simulink model "LaneFollowingTestBenchExample"  (R2023a)
settings: Solver=VariableStepAuto  StartTime=0.0  StopTime=simStopTime  RelTol=1e-3
PostLoadFcn:
  | if exist('scenarioName','var')
  |   helperLFSetUp(scenarioName)
  | else
  |   helperLFSetUp()
  | end
values from neighbouring files (symbols this model uses):
  Ts = 0.01    [Working.m]    (also in Working_flipped.m)
  v_set = 15    [helperLFSetUp.m]
undefined symbols (not defined in the file or in its folder): driving, egoCarID, lr, m, matlabshared, tau
libraries: drivingscenarioandsensors x6, trackingutilitieslib x1, autolibshared x1
CloseFcn:
  | helperLFCleanUp
settings Model: Creator=The MathWorks, Inc.  LastModifiedBy=Administrator
settings SolverCC: AlgebraicLoopSolver=TrustRegion
settings DataIOCC: ReturnWorkspaceOutputs=off
settings DebuggingCC: ParameterPrecisionLossMsg=none  UnconnectedInputMsg=warning  UnconnectedOutputMsg=warning  UnconnectedLineMsg=warning  PregeneratedLibrarySubsystemCodeDiagnostic=none  ArithmeticOperatorsInVariantConditions=warning
settings HardwareCC: ProdLongLongMode=on
settings ModelReferenceCC: EnableRefExpFcnMdlSchedulingChecks=on
settings SFSimCC: SimUseLocalCustomCode=off
settings RTWCC: GenerateReport=on  RTWUseLocalCustomCode=off  LaunchReport=on  DLArmComputeVersion=19.05
settings ConfigComp: CovScope=ReferencedModels  CovIncludeTopModel=off

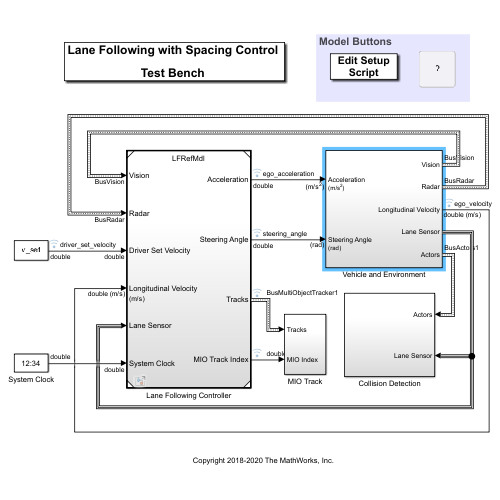
[thumbnail: Simulink's stored preview of the top-level diagram]
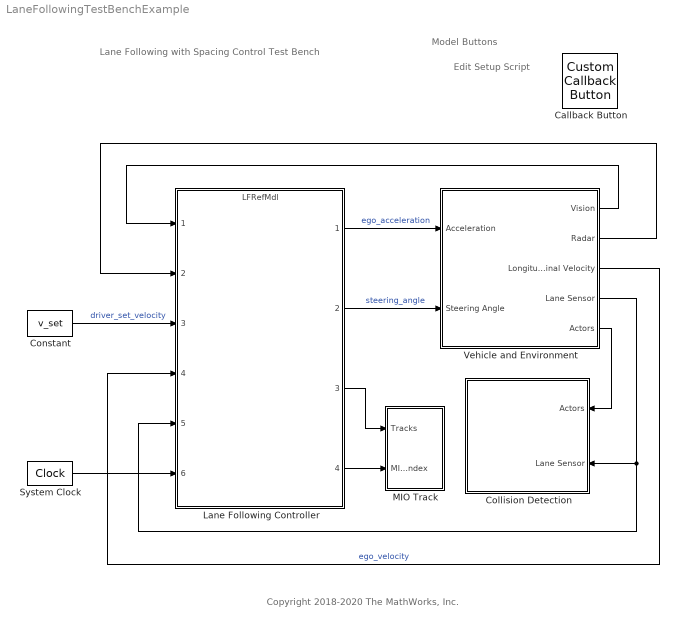
== system LaneFollowingTestBenchExample ==
  note: Copyright 2018-2020 The MathWorks, Inc.
  note: Edit Setup Script
  note: Lane Following with Spacing Control
      | Test Bench
  note: Model Buttons
  Callback Button : CustomCallbackButton  Configuration="{\"components\":[{\"name\":\"BackgroundImageComponent\",\"settings\":{\"image\":{\"size\":[0,0],\"src\":\"default\",\"srcOrientation\":\"Right\"},\"position\":[0,0,1,1]}},{\"name\":\"ButtonStateComponent\",\"settings\":{\"buttonType\":\"momentary\",\"clickFcn\":\"exampleName = 'lane-following-control-with-sensor-fusion-and-lane-detection.html';\\nif license('test','automated_driving_toolbox') && ~isempty(ver('driving'))\\n   web(fullfile(docroot,'driving','ug', exampleName));\\nelseif license('test','MPC_Toolbox') && ~isempty(ver('mpc'))\\n    web(fullfile(docroot,'mpc','ug', exampleName));\\nelse\\n    web(fullfile('https:\\/\\/www.mathworks.com\\/help','driving','ug',exampleName));\\nend\",\"onValue\":1,\"position\":[0,0,1,1],\"pressDelay\":\"500\",\"pressFcn\":\"\",\"repeatInterval\":\"0\",\"states\":[{\"horizontalAlignment\":\"center\",\"image\":{\"position\":[0,0,1,1],\"src\":\"default\",\"srcOrientation\":\"Right\"},\"label\":{\"color\":[0.01176470588,0.01176470588,0.01176470588,1],\"icon\":{\"size\":[0,0],\"src\":\"default\",\"srcOrientation\":\"Right\"},\"iconPlacement\":\"left\",\"text\":{\"content\":\"?\"}},\"labelOffset\":[0,0],\"verticalAlignment\":\"middle\"},{\"horizontalAlignment\":\"center\",\"image\":{\"position\":[0,0,1,1],\"src\":\"default\",\"srcOrientation\":\"Right\"},\"label\":{\"color\":[0.01176470588,0.01176470588,0.01176470588,1],\"icon\":{\"size\":[0,0],\"src\":\"default\",\"srcOrientation\":\"Right\"},\"iconPlacement\":\"left\",\"text\":{\"content\":\"?\"}},\"labelOffset\":[0,0],\"verticalAlignment\":\"middle\"},{\"horizontalAlignment\":\"center\",\"image\":{\"position\":[0,0,1,1],\"src\":\"default\",\"srcOrientation\":\"Right\"},\"label\":{\"color\":[0.01176470588,0.01176470588,0.01176470588,1],\"icon\":{\"size\":[0,0],\"src\":\"default\",\"srcOrientation\":\"Right\"},\"iconPlacement\":\"left\",\"text\":{\"content\":\"?\"}},\"labelOffset\":[0,0],\"verticalAlignment\":\"middle\"},{\"horizontalAlignment\":\"center\",\"image\":{\"position\":[0,0,1,1],\"src\":\"default\",\"srcOrientation\":\"Right\"},\"label\":{\"color\":[0.01176470588,0.01176470588,0.01176470588,1],\"icon\":{\"size\":[0,0],\"src\":\"default\",\"srcOrientation\":\"Right\"},\"iconPlacement\":\"left\",\"text\":{\"content\":\"?\"}},\"labelOffset\":[0,0],\"verticalAlignment\":\"middle\"}]}},{\"name\":\"ForegroundImageComponent\",\"settings\":{\"image\":{\"size\":[0,0],\"src\":\"default\",\"srcOrientation\":\"Right\"},\"isForeground\":1,\"position\":[0,0,1,1]}}],\"settings\":{\"BindingType\":\"standalone\",\"backgroundColor\":[244,244,244,1],\"backgroundOffset\":0.2,\"backgroundOpacity\":1,\"fixedAspectRatio\":\"off\",\"foregroundColor\":[0.01176470588,0.01176470588,0.01176470588,1],\"migratedFromLegacy\":true,\"useBackgroundColor\":true,\"variant\":\"callback\",\"version\":\"R2023a\"},\"type\":\"Button\"}"  CustomBackgroundColor="{\"color\":[0.9568627451,0.9568627451,0.9568627451],\"show\":true}"
  Collision Detection : Subsystem
  Constant : Constant  Value=v_set  SampleTime=Ts
  Lane Following Controller : ModelReference  ModelNameDialog=LFRefMdl  SimulationMode=Normal  CodeInterface=Top model  ModelReferenceVersion=6.1
  MIO Track : Subsystem
  System Clock : DigitalClock  SampleTime=Ts
  Vehicle and Environment : Subsystem
  wires:
  Lane Following Controller/1 -> Vehicle and Environment/1(Acceleration)  "ego_acceleration"
  Lane Following Controller/2 -> Vehicle and Environment/2(Steering Angle)  "steering_angle"
  Constant/1 -> Lane Following Controller/3  "driver_set_velocity"
  Vehicle and Environment/3(Longitudinal Velocity) -> Lane Following Controller/4  "ego_velocity"
  Vehicle and Environment/4(Lane Sensor) -> Lane Following Controller/5, Collision Detection/2(Lane Sensor)
  Vehicle and Environment/2(Radar) -> Lane Following Controller/2
  Vehicle and Environment/1(Vision) -> Lane Following Controller/1
  Lane Following Controller/3 -> MIO Track/1(Tracks)
  Lane Following Controller/4 -> MIO Track/2(MIO Index)
  Vehicle and Environment/5(Actors) -> Collision Detection/1(Actors)
  System Clock/1 -> Lane Following Controller/6

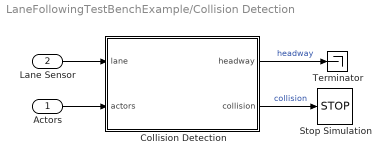
== system LaneFollowingTestBenchExample/Collision Detection ==
  Actors : Inport
  Lane Sensor : Inport  Port=2
  Collision Detection : MATLAB Function  TreatAsAtomicUnit=on
  Stop Simulation : Stop
  Terminator : Terminator
  wires:
  Collision Detection/2(collision) -> Stop Simulation/1  "collision"
  Actors/1 -> Collision Detection/2(actors)
  Lane Sensor/1 -> Collision Detection/1(lane)
  Collision Detection/1(headway) -> Terminator/1  "headway"

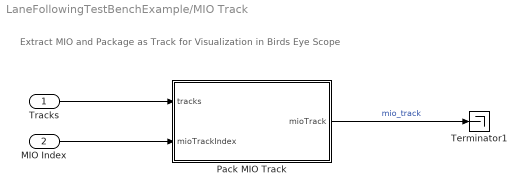
== system LaneFollowingTestBenchExample/MIO Track ==
  note: Extract MIO and Package as Track for Visualization in Birds Eye Scope
  Tracks : Inport
  MIO Index : Inport  Port=2
  Pack MIO Track : MATLAB Function  TreatAsAtomicUnit=on
  Terminator1 : Terminator
  wires:
  Tracks/1 -> Pack MIO Track/1(tracks)
  Pack MIO Track/1(mioTrack) -> Terminator1/1  "mio_track"
  MIO Index/1 -> Pack MIO Track/2(mioTrackIndex)

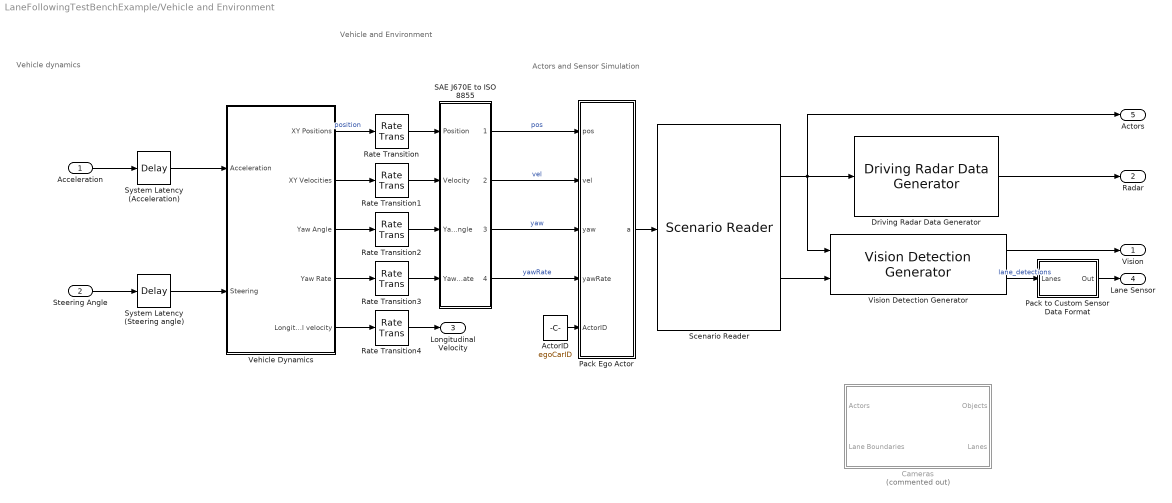
== system LaneFollowingTestBenchExample/Vehicle and Environment ==
  note: Vehicle dynamics
  note: Actors and Sensor Simulation
  note: Vehicle and Environment
  Acceleration : Inport  Unit=m/s^2
  Steering Angle : Inport  Port=2  Unit=rad
  ActorID : Constant  Value=egoCarID
  Cameras : Subsystem  Commented=on
  Driving Radar Data Generator : drivingscenarioandsensors/Driving Radar Data Generator  SensorIndex=2  UpdateRate=10  MountingLocation=[ 3.7, 0, 0.2 ]  MountingAngles=[0 0 0]  HasElevation=off  HasRangeRate=on  HasNoise=on  HasFalseAlarms=on  HasOcclusion=on  MaxNumReportsSource=Property  MaxNumReports=50  TargetReportFormat=Clustered detections  DetectionCoordinates=Body  TrackCoordinates=Body  BusNameSource=Property  BusName=BusRadar  AzimuthResolution=4  ElevationResolution=5  RangeResolution=2.5  RangeRateResolution=0.5  AzimuthBiasFraction=0.1  ElevationBiasFraction=0.1  RangeBiasFraction=0.05  RangeRateBiasFraction=0.05  FieldOfView=[ 20, 5 ]  RangeLimits=[ 0, 174 ]  RangeRateLimits=[ -100, 100 ]  DetectionProbability=0.9  FalseAlarmRate=1e-06  ReferenceRange=100  ReferenceRCS=0  CenterFrequency=77e9  FilterInitializationFcn=initcvekf  ConfirmationThreshold=[2 3]  DeletionThreshold=[5 5]  InitialSeedSource=Repeatable  InitialSeed=0  UsedSeed=matlabshared.tracking.internal.SimulinkUtilities.seedManager(gcb)  ProfilesSource=From Scenario Reader block  ProfilesParameters=driving.internal.ActorProfilesRadarParameters  ProfilesExpression=struct('ClassID',0,'Length',4.7,'Width',1.8,'Height',1.4,'OriginOffset',[-1.35 0 0],'RCSPattern',[10 10;10 10],'RCSAzimuthAngles',[-180 180],'RCSElevationAngles',[-90 90])
  Pack Ego Actor : MATLAB Function  TreatAsAtomicUnit=on
  Pack to Custom Sensor Data Format : Subsystem
  Rate Transition{,1..4} (5 alike) : RateTransition  OutPortSampleTime=Ts
  SAE J670E to ISO 8855 : Subsystem
  Scenario Reader : drivingscenarioandsensors/Scenario Reader  ScenarioSource=From workspace  ScenarioFileName=LFACC_04_Curve_CutInOut.mat  ScenarioVariableName=scenario  OutputCoordinateSystem=Vehicle coordinates  EgoVehicleSource=Input port  EgoVehicleActorID=egoCarID  OrientVehiclesOnRoad=off  OutputEgoVehiclePose=off  OutputEgoVehicleState=off  SampleTime=0.1  LaneBoundaryOutput=Ego vehicle lane boundaries  LaneBoundaryDistance=0:0.5:60  LaneBoundaryLocation=Inner edge of lane markings  BusNameSource=Auto  BusName=BusActors  BusNumActorsSource=Scenario  BusNumActors=100  BusName2Source=Auto  BusName2=BusLaneBoundaries  BusNumLaneBoundariesSource=Scenario  BusNumLaneBoundaries=10  BusName3Source=Auto  BusName3=BusEgoActor  BusName4Source=Auto  BusName4=BusEgoState  ShowCoordinateLabels=on  SimulateUsing=Interpreted execution
  System Latency (Acceleration) : TransportDelay  DelayTime=Ts
  System Latency (Steering angle) : TransportDelay  DelayTime=Ts
  Vehicle Dynamics : Subsystem  VariantControl=Variant2
  Vision Detection Generator : drivingscenarioandsensors/Vision Detection Generator  SensorIndex=1  DetectorOutput=Lanes and objects  UpdateInterval=0.1  LaneUpdateInterval=0.1  SensorLocation=[ 1.9, 0 ]  Height=1.1  Yaw=0  Pitch=1  Roll=0  BusNameSource=Property  BusName=BusVision  BusName2Source=Property  BusName2=BusLanes  MaxNumDetectionsSource=Property  MaxNumDetections=20  MaxNumLanesSource=Property  MaxNumLanes=2  DetectionCoordinates=Ego Cartesian  SimulateUsing=Interpreted execution  MaxRange=150  BoundingBoxAccuracy=5  ProcessNoiseIntensity=5  MaxSpeed=50  MaxAllowedOcclusion=0.5  MinObjectImageSize=[ 10, 10 ]  DetectionProbability=0.9  FalsePositivesPerImage=0.1  MinLaneImageSize=[ 20, 3 ]  LaneBoundaryAccuracy=3  HasNoise=on  InitialSeedSource=Repeatable  InitialSeed=0  UsedSeed=driving.internal.SimulinkUtilities.seedManager(gcb)  ActorProfilesSource=From Scenario Reader block  ActorProfilesParameters=driving.internal.ActorProfilesParameters  ActorProfilesExpression=struct( 'ClassID', 0, 'Length', 4.7, 'Width', 1.8, 'Height', 1.4, 'OriginOffset', [ -1.35, 0, 0 ] )  Intrinsics=driving.internal.cameraIntrinsics('FocalLength',[ 600,600 ])
  Vision : Outport  VectorParamsAs1DForOutWhenUnconnected=off
  Radar : Outport  Port=2  VectorParamsAs1DForOutWhenUnconnected=off
  Longitudinal Velocity : Outport  Port=3  VectorParamsAs1DForOutWhenUnconnected=off
  Lane Sensor : Outport  Port=4  VectorParamsAs1DForOutWhenUnconnected=off
  Actors : Outport  Port=5  VectorParamsAs1DForOutWhenUnconnected=off
  wires:
  Scenario Reader/1 -> Actors/1, Driving Radar Data Generator/1, Vision Detection Generator/1
  Vehicle Dynamics/2(XY Velocities) -> Rate Transition1/1
  Vehicle Dynamics/3(Yaw Angle) -> Rate Transition2/1
  Vehicle Dynamics/4(Yaw Rate) -> Rate Transition3/1
  Vehicle Dynamics/1(XY Positions) -> Rate Transition/1  "position"
  Pack to Custom Sensor Data Format/1(Out) -> Lane Sensor/1
  Rate Transition4/1 -> Longitudinal Velocity/1
  Vehicle Dynamics/5(Longitudinal velocity) -> Rate Transition4/1
  Scenario Reader/2 -> Vision Detection Generator/2
  Driving Radar Data Generator/1 -> Radar/1
  Pack Ego Actor/1(a) -> Scenario Reader/1
  Acceleration/1 -> System Latency (Acceleration)/1
  Steering Angle/1 -> System Latency (Steering angle)/1
  System Latency (Acceleration)/1 -> Vehicle Dynamics/1(Acceleration)
  System Latency (Steering angle)/1 -> Vehicle Dynamics/2(Steering)
  SAE J670E to ISO 8855/1(1) -> Pack Ego Actor/1(pos)  "pos"
  SAE J670E to ISO 8855/2(2) -> Pack Ego Actor/2(vel)  "vel"
  SAE J670E to ISO 8855/3(3) -> Pack Ego Actor/3(yaw)  "yaw"
  SAE J670E to ISO 8855/4(4) -> Pack Ego Actor/4(yawRate)  "yawRate"
  Rate Transition3/1 -> SAE J670E to ISO 8855/4(Yaw Rate)
  Rate Transition2/1 -> SAE J670E to ISO 8855/3(Yaw Angle)
  Rate Transition1/1 -> SAE J670E to ISO 8855/2(Velocity)
  Rate Transition/1 -> SAE J670E to ISO 8855/1(Position)
  ActorID/1 -> Pack Ego Actor/5(ActorID)
  Vision Detection Generator/2 -> Pack to Custom Sensor Data Format/1(Lanes)  "lane_detections"
  Vision Detection Generator/1 -> Vision/1

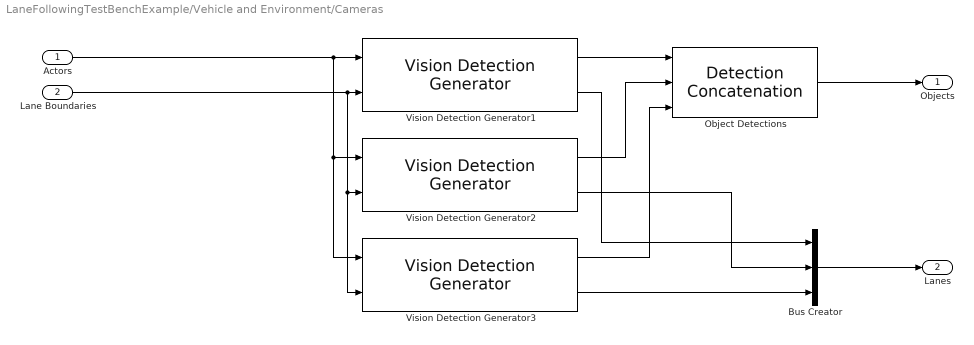
== system LaneFollowingTestBenchExample/Vehicle and Environment/Cameras ==
  Actors : Inport
  Lane Boundaries : Inport  Port=2
  Bus Creator : BusCreator  Inputs=3
  Object Detections : trackingutilitieslib/Detection Concatenation  NumInputs=3  BusNameSource=Auto  BusName=BusDetectionConcatenation  SimulateUsing=Interpreted execution
      settings: LibrarySourceBlock=drivinglib/Detection Concatenation
  Vision Detection Generator1 : drivingscenarioandsensors/Vision Detection Generator  SensorIndex=3  DetectorOutput=Lanes and objects  UpdateInterval=0.1  LaneUpdateInterval=0.1  SensorLocation=[ 1.835, 0 ]  Height=1.1  Yaw=0  Pitch=1  Roll=0  BusNameSource=Property  BusName=BusVision  BusName2Source=Property  BusName2=BusLanes  MaxNumDetectionsSource=Property  MaxNumDetections=20  MaxNumLanesSource=Property  MaxNumLanes=2  DetectionCoordinates=Ego Cartesian  SimulateUsing=Interpreted execution  MaxRange=150  BoundingBoxAccuracy=5  ProcessNoiseIntensity=5  MaxSpeed=50  MaxAllowedOcclusion=0.5  MinObjectImageSize=[ 10, 10 ]  DetectionProbability=0.9  FalsePositivesPerImage=0.1  MinLaneImageSize=[ 20, 3 ]  LaneBoundaryAccuracy=3  HasNoise=on  InitialSeedSource=Repeatable  InitialSeed=0  UsedSeed=driving.internal.SimulinkUtilities.seedManager(gcb)  ActorProfilesSource=From Scenario Reader block  ActorProfilesParameters=driving.internal.ActorProfilesParameters  ActorProfilesExpression=struct( 'ClassID', 0, 'Length', 4.7, 'Width', 1.8, 'Height', 1.4, 'OriginOffset', [ -1.35, 0, 0 ] )  Intrinsics=driving.internal.cameraIntrinsics('FocalLength',[ 800,800 ])
  Vision Detection Generator2 : drivingscenarioandsensors/Vision Detection Generator  SensorIndex=5  DetectorOutput=Lanes and objects  UpdateInterval=0.1  LaneUpdateInterval=0.1  SensorLocation=[2, 0.945]  Height=1.1  Yaw=90  Pitch=1  Roll=0  BusNameSource=Property  BusName=BusVision  BusName2Source=Property  BusName2=BusLanes  MaxNumDetectionsSource=Property  MaxNumDetections=20  MaxNumLanesSource=Property  MaxNumLanes=2  DetectionCoordinates=Ego Cartesian  SimulateUsing=Interpreted execution  MaxRange=150  BoundingBoxAccuracy=5  ProcessNoiseIntensity=5  MaxSpeed=50  MaxAllowedOcclusion=0.5  MinObjectImageSize=[ 10, 10 ]  DetectionProbability=0.9  FalsePositivesPerImage=0.1  MinLaneImageSize=[ 20, 3 ]  LaneBoundaryAccuracy=3  HasNoise=on  InitialSeedSource=Repeatable  InitialSeed=0  UsedSeed=driving.internal.SimulinkUtilities.seedManager(gcb)  ActorProfilesSource=From Scenario Reader block  ActorProfilesParameters=driving.internal.ActorProfilesParameters  ActorProfilesExpression=struct( 'ClassID', 0, 'Length', 4.7, 'Width', 1.8, 'Height', 1.4, 'OriginOffset', [ -1.35, 0, 0 ] )  Intrinsics=driving.internal.cameraIntrinsics('FocalLength',[ 800,800 ])
  Vision Detection Generator3 : drivingscenarioandsensors/Vision Detection Generator  SensorIndex=4  DetectorOutput=Lanes and objects  UpdateInterval=0.1  LaneUpdateInterval=0.1  SensorLocation=[ 2, -0.945 ]  Height=1.1  Yaw=-90  Pitch=1  Roll=0  BusNameSource=Property  BusName=BusVision  BusName2Source=Property  BusName2=BusLanes  MaxNumDetectionsSource=Property  MaxNumDetections=20  MaxNumLanesSource=Property  MaxNumLanes=2  DetectionCoordinates=Ego Cartesian  SimulateUsing=Interpreted execution  MaxRange=150  BoundingBoxAccuracy=5  ProcessNoiseIntensity=5  MaxSpeed=50  MaxAllowedOcclusion=0.5  MinObjectImageSize=[ 10, 10 ]  DetectionProbability=0.9  FalsePositivesPerImage=0.1  MinLaneImageSize=[ 20, 3 ]  LaneBoundaryAccuracy=3  HasNoise=on  InitialSeedSource=Repeatable  InitialSeed=0  UsedSeed=driving.internal.SimulinkUtilities.seedManager(gcb)  ActorProfilesSource=From Scenario Reader block  ActorProfilesParameters=driving.internal.ActorProfilesParameters  ActorProfilesExpression=struct( 'ClassID', 0, 'Length', 4.7, 'Width', 1.8, 'Height', 1.4, 'OriginOffset', [ -1.35, 0, 0 ] )  Intrinsics=driving.internal.cameraIntrinsics('FocalLength',[ 800,800 ])
  Objects : Outport
  Lanes : Outport  Port=2
  wires:
  Actors/1 -> Vision Detection Generator1/1, Vision Detection Generator2/1, Vision Detection Generator3/1
  Lane Boundaries/1 -> Vision Detection Generator3/2, Vision Detection Generator2/2, Vision Detection Generator1/2
  Vision Detection Generator1/1 -> Object Detections/1
  Vision Detection Generator2/1 -> Object Detections/2
  Vision Detection Generator2/2 -> Bus Creator/2
  Vision Detection Generator3/1 -> Object Detections/3
  Vision Detection Generator3/2 -> Bus Creator/3
  Vision Detection Generator1/2 -> Bus Creator/1
  Object Detections/1 -> Objects/1
  Bus Creator/1 -> Lanes/1

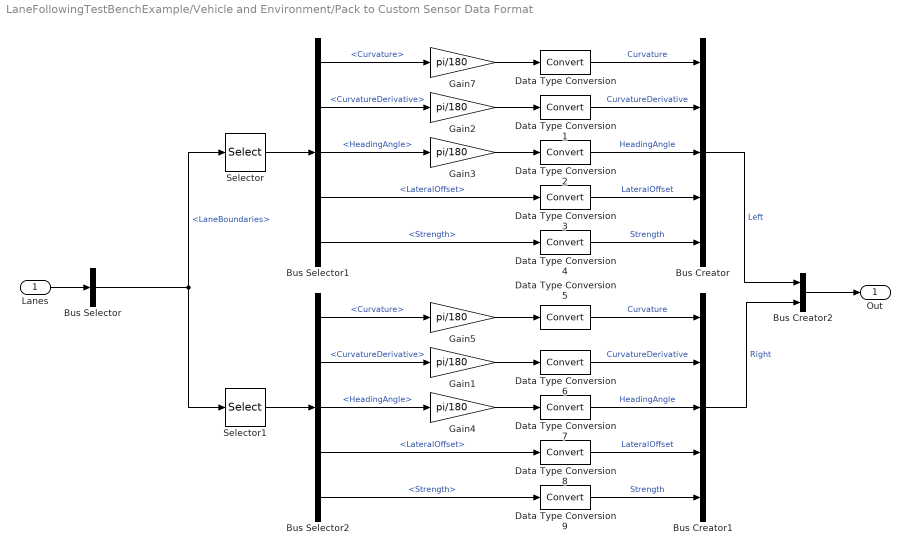
== system LaneFollowingTestBenchExample/Vehicle and Environment/Pack to Custom Sensor Data Format ==
  Lanes : Inport
  Bus Creator : BusCreator  Inputs=5  OutDataTypeStr=Bus: LaneSensorBoundaries
  Bus Creator1 : BusCreator  Inputs=5  OutDataTypeStr=Bus: LaneSensorBoundaries
  Bus Creator2 : BusCreator  Inputs=2  OutDataTypeStr=Bus: LaneSensor
  Bus Selector : BusSelector  OutputSignals=LaneBoundaries
  Bus Selector1 : BusSelector  OutputSignals=Curvature,CurvatureDerivative,HeadingAngle,LateralOffset,Strength
  Bus Selector2 : BusSelector  OutputSignals=Curvature,CurvatureDerivative,HeadingAngle,LateralOffset,Strength
  Data Type Conversion{,1..9} (10 alike) : DataTypeConversion  SaturateOnIntegerOverflow=off  RndMeth=Floor
  Gain{1..5,7} (6 alike) : Gain  Gain=pi/180
  Selector : Selector  InputPortWidth=2  IndexOptions=Index vector (dialog)  Indices=1  OutputSizes=1
  Selector1 : Selector  InputPortWidth=2  IndexOptions=Index vector (dialog)  Indices=2  OutputSizes=1
  Out : Outport  VectorParamsAs1DForOutWhenUnconnected=off
  wires:
  Lanes/1 -> Bus Selector/1
  Bus Selector/1 -> Selector/1, Selector1/1  "<LaneBoundaries>"
  Selector/1 -> Bus Selector1/1
  Bus Selector1/2 -> Gain2/1  "<CurvatureDerivative>"
  Bus Selector1/1 -> Gain7/1  "<Curvature>"
  Bus Selector1/3 -> Gain3/1  "<HeadingAngle>"
  Gain7/1 -> Data Type Conversion/1
  Gain2/1 -> Data Type Conversion1/1
  Gain3/1 -> Data Type Conversion2/1
  Bus Selector1/4 -> Data Type Conversion3/1  "<LateralOffset>"
  Bus Selector1/5 -> Data Type Conversion4/1  "<Strength>"
  Data Type Conversion/1 -> Bus Creator/1  "Curvature"
  Data Type Conversion1/1 -> Bus Creator/2  "CurvatureDerivative"
  Data Type Conversion2/1 -> Bus Creator/3  "HeadingAngle"
  Data Type Conversion3/1 -> Bus Creator/4  "LateralOffset"
  Data Type Conversion4/1 -> Bus Creator/5  "Strength"
  Data Type Conversion9/1 -> Bus Creator1/5  "Strength"
  Data Type Conversion6/1 -> Bus Creator1/2  "CurvatureDerivative"
  Data Type Conversion7/1 -> Bus Creator1/3  "HeadingAngle"
  Data Type Conversion8/1 -> Bus Creator1/4  "LateralOffset"
  Data Type Conversion5/1 -> Bus Creator1/1  "Curvature"
  Bus Selector2/1 -> Gain5/1  "<Curvature>"
  Selector1/1 -> Bus Selector2/1
  Bus Selector2/4 -> Data Type Conversion8/1  "<LateralOffset>"
  Bus Selector2/5 -> Data Type Conversion9/1  "<Strength>"
  Bus Selector2/2 -> Gain1/1  "<CurvatureDerivative>"
  Gain4/1 -> Data Type Conversion7/1
  Gain5/1 -> Data Type Conversion5/1
  Gain1/1 -> Data Type Conversion6/1
  Bus Selector2/3 -> Gain4/1  "<HeadingAngle>"
  Bus Creator2/1 -> Out/1
  Bus Creator/1 -> Bus Creator2/1  "Left"
  Bus Creator1/1 -> Bus Creator2/2  "Right"

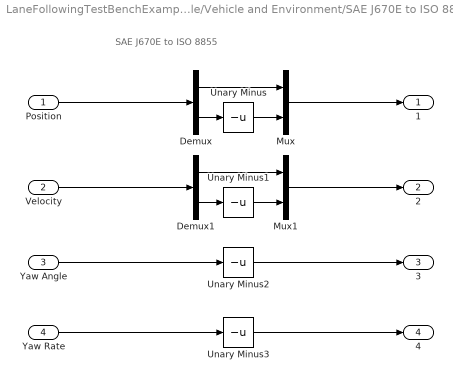
== system LaneFollowingTestBenchExample/Vehicle and Environment/SAE J670E to ISO 8855 ==
  note: SAE J670E to ISO 8855
  Position : Inport  Unit=m
  Velocity : Inport  Port=2  Unit=m/s
  Yaw Angle : Inport  Port=3  Unit=deg
  Yaw Rate : Inport  Port=4  Unit=deg/s
  Demux : Demux  Outputs=2
  Demux1 : Demux  Outputs=2
  Mux : Mux  Inputs=2
  Mux1 : Mux  Inputs=2
  Unary Minus{,1..3} (4 alike) : UnaryMinus
  1 : Outport  VectorParamsAs1DForOutWhenUnconnected=off
  2 : Outport  Port=2  VectorParamsAs1DForOutWhenUnconnected=off
  3 : Outport  Port=3  VectorParamsAs1DForOutWhenUnconnected=off
  4 : Outport  Port=4  VectorParamsAs1DForOutWhenUnconnected=off
  wires:
  Yaw Rate/1 -> Unary Minus3/1
  Yaw Angle/1 -> Unary Minus2/1
  Demux/1 -> Mux/1
  Demux/2 -> Unary Minus/1
  Unary Minus/1 -> Mux/2
  Unary Minus1/1 -> Mux1/2
  Demux1/2 -> Unary Minus1/1
  Demux1/1 -> Mux1/1
  Mux1/1 -> 2/1
  Mux/1 -> 1/1
  Position/1 -> Demux/1
  Velocity/1 -> Demux1/1
  Unary Minus2/1 -> 3/1
  Unary Minus3/1 -> 4/1

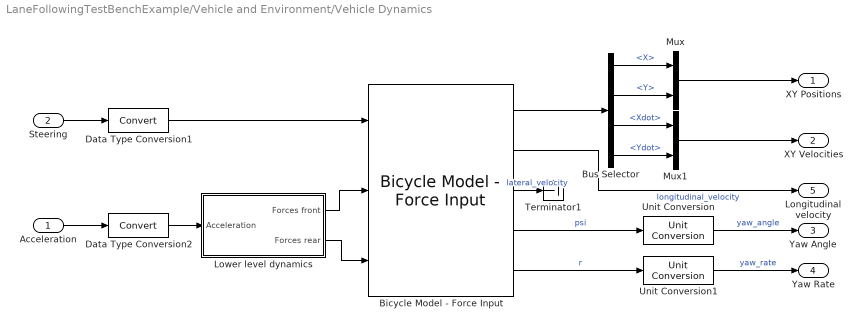
== system LaneFollowingTestBenchExample/Vehicle and Environment/Vehicle Dynamics ==
  Acceleration : Inport  Unit=m/s^2
  Steering : Inport  Port=2  Unit=rad
  Bicycle Model - Force Input : autolibshared/Bicycle Model - Force Input  trackMode=Single (bicycle)  inputMode=External longitudinal forces  frontSteerMode=on  rearSteerMode=off  windMode=off  muMode=off  extFMode=off  extMMode=off  aMode=3  NF=2  NR=2  m=m  a=lf  b=lr  h=0.35  X_o=x0_ego  xdot_o=v0_ego  CalphaMode=off  sigmaMode=on  w=[1.4,1.4]  Cy_f=Cf  Cy_r=Cr  sigma_f=.1  sigma_r=.1  alpha_f_brk=[-.1 .1]  Cy_f_data=[-9e3 9e3]  alpha_r_brk=[-.1 .1]  Cy_r_data=[-9e3 9e3]  Y_o=y0_ego  ydot_o=0  Izz=Iz  psi_o=yaw0_ego  r_o=0  Af=0  Cd=.3  Cl=.1  Cpm=.1  beta_w=[0:0.01:0.3]  Cs=[0:0.03:0.9]  Cym=[0:0.01:0.3]  Pabs=101325  Tair=273  g=9.81  mu=1  xdot_tol=.01  Fznom=5000  Fxtire_sat=1e6  Fytire_sat=1e6  longOff=0  latOff=0  vertOff=0
  Bus Selector : BusSelector  OutputSignals=InertFrm.FrntAxl.Disp.X,InertFrm.FrntAxl.Disp.Y,InertFrm.FrntAxl.Vel.Xdot,InertFrm.FrntAxl.Vel.Ydot
  Data Type Conversion1 : DataTypeConversion  SaturateOnIntegerOverflow=off  RndMeth=Floor
  Data Type Conversion2 : DataTypeConversion  SaturateOnIntegerOverflow=off  RndMeth=Floor
  Lower level dynamics : Subsystem
  Mux : Mux  Inputs=2
  Mux1 : Mux  Inputs=2
  Terminator1 : Terminator
  Unit Conversion : UnitConversion  OutputType=Inherit: Inherit via back propagation
  Unit Conversion1 : UnitConversion  OutputType=Inherit: Inherit via back propagation
  XY Positions : Outport  Unit=m  VectorParamsAs1DForOutWhenUnconnected=off
  XY Velocities : Outport  Port=2  Unit=m/s  VectorParamsAs1DForOutWhenUnconnected=off
  Yaw Angle : Outport  Port=3  Unit=deg  VectorParamsAs1DForOutWhenUnconnected=off
  Yaw Rate : Outport  Port=4  Unit=degree/s  VectorParamsAs1DForOutWhenUnconnected=off
  Longitudinal velocity : Outport  Port=5  VectorParamsAs1DForOutWhenUnconnected=off
  wires:
  Lower level dynamics/2(Forces rear) -> Bicycle Model - Force Input/3
  Lower level dynamics/1(Forces front) -> Bicycle Model - Force Input/2
  Data Type Conversion2/1 -> Lower level dynamics/1(Acceleration)
  Data Type Conversion1/1 -> Bicycle Model - Force Input/1
  Acceleration/1 -> Data Type Conversion2/1
  Steering/1 -> Data Type Conversion1/1
  Bus Selector/1 -> Mux/1  "<X>"
  Unit Conversion/1 -> Yaw Angle/1  "yaw_angle"
  Bicycle Model - Force Input/5 -> Unit Conversion1/1  "r"
  Bus Selector/4 -> Mux1/2  "<Ydot>"
  Bicycle Model - Force Input/4 -> Unit Conversion/1  "psi"
  Bus Selector/2 -> Mux/2  "<Y>"
  Bicycle Model - Force Input/2 -> Longitudinal velocity/1  "longitudinal_velocity"
  Bus Selector/3 -> Mux1/1  "<Xdot>"
  Bicycle Model - Force Input/1 -> Bus Selector/1
  Bicycle Model - Force Input/3 -> Terminator1/1  "lateral_velocity"
  Mux/1 -> XY Positions/1
  Mux1/1 -> XY Velocities/1
  Unit Conversion1/1 -> Yaw Rate/1  "yaw_rate"

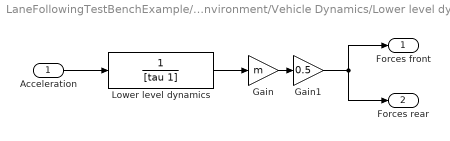
== system LaneFollowingTestBenchExample/Vehicle and Environment/Vehicle Dynamics/Lower level dynamics ==
  Acceleration : Inport
  Gain : Gain  Gain=m
  Gain1 : Gain  Gain=0.5
  Lower level dynamics : TransferFcn  Denominator=[tau 1]
  Forces front : Outport  VectorParamsAs1DForOutWhenUnconnected=off
  Forces rear : Outport  Port=2  VectorParamsAs1DForOutWhenUnconnected=off
  wires:
  Gain/1 -> Gain1/1
  Gain1/1 -> Forces front/1, Forces rear/1
  Acceleration/1 -> Lower level dynamics/1
  Lower level dynamics/1 -> Gain/1

== matlab function LaneFollowingTestBenchExample/Collision Detection/Collision Detection ==
  data: lane input; headway output; actors input; collision output
function [headway,collision] = collisionDetect(lane, actors)

% If lane detection is not available, the ego car is assumed to be located
% in the middle of its lane. The lane width is assumed to be 3.6m, typical
% highway lane width.
laneWidth = 3.6;
halfLaneWidth = laneWidth/2;

% left lane
if lane.Left.Strength > 0.01
    lb = [lane.Left.CurvatureDerivative/6,...
        lane.Left.Curvature/2,...
        lane.Left.HeadingAngle,...
        lane.Left.LateralOffset];
else
    lb = single([0,0,0,halfLaneWidth]);
end

% right lane
if lane.Right.Strength > 0.01
    rb = [lane.Right.CurvatureDerivative/6,...
        lane.Right.Curvature/2,...
        lane.Right.HeadingAngle,...
        lane.Right.LateralOffset];
else
    rb = single([0,0,0,-halfLaneWidth]);    
end

dist = zeros(1,actors.NumActors);

for i = 1:actors.NumActors
    x = actors.Actors(i).Position(1);
    y = actors.Actors(i).Position(2);
    
    yleftLane  = polyval(lb,x);
    yrightLane = polyval(rb,x);
    
    if (yrightLane <= y) && (y <= yleftLane) % within lane boundary?
        dist(i) = hypot(x,y); 
    else
        dist(i) = 100;
    end       
end

headway = min(dist) - 4.7;  % headway from the lead vehicle's trailing surface to the ego vehicle's leading surface
if headway < 1.5
    collision = true; % collision detected
else
    collision = false;
end

== matlab function LaneFollowingTestBenchExample/MIO Track/Pack MIO Track ==
  data: tracks input; mioTrack output Bus: BusMultiObjectTracker1; mioTrackIndex input
function mioTrack = fcn(tracks, mioTrackIndex)
% Extract MIO track and package for visualization in Birds Eye Scope

mioTrack = tracks;

if mioTrackIndex > 0
    % First track represents MIO
    mioTrack.NumTracks = 1;
    mioTrack.Tracks(1) = tracks.Tracks(mioTrackIndex);
else
    % No valid MIO track
    mioTrack.NumTracks = 0;
end

== matlab function LaneFollowingTestBenchExample/Vehicle and Environment/Pack Ego Actor ==
  data: pos input; a output Bus: BusActors1Actors size=1; vel input; yaw input; yawRate input; ActorID input
function a = packEgo(pos,vel,yaw,yawRate,ActorID)
% Pack ego information into a single ego actor bus
%
% Imoprtant note:
% Output is a bus of type BusActorsActors. This is the same bus used by the
% Scenario Reader to output an individual actor. If you change the
% output bus name of Scenario Reader change the output bus name here
% as well by clicking on 'Edit Data' in the menu above.

a = struct(...
    'ActorID',ActorID,...
    'Position', [pos(1) pos(2) 0], ...
    'Velocity', [vel(1) vel(2) 0], ...
    'Roll', 0, ...
    'Pitch', 0, ...
    'Yaw', yaw, ...
    'AngularVelocity', [0 0 yawRate]);
